simulink subsystem "Luenberger_Tower_FA_Observer"  (R2021a)
settings: Solver=VariableStepAuto  StartTime=0.0  StopTime=10.0  RelTol=1e-3
values from neighbouring files (symbols this model uses):
  Parameters =     [Parameters.mat]
undefined symbols (not defined in the file or in its folder): luenGainDisc1, sys_tower_fa_d_obsv1
libraries: dspstat3 x2
settings Model: Creator=atindriyopamos  LastModifiedBy=zfeng1

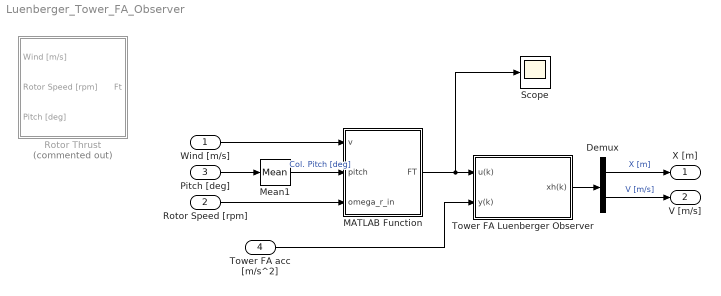
== system Luenberger_Tower_FA_Observer ==
  Wind [m/s] : Inport
  Rotor Speed [rpm] : Inport  Port=2
  Pitch [deg] : Inport  Port=3
  Tower FA acc [m/s^2] : Inport  Port=4
  Demux : Demux  Outputs=2
  MATLAB Function : MATLAB Function  TreatAsAtomicUnit=on
  Mean1 : dspstat3/Mean  run=off  InputProcessing=Columns as channels (frame based)  reset_popup=None  directionMode=Entire input  dimension=1  roiEnable=off  roiType=Rectangles  roiPortion=Entire ROI  roiOutput=Individual statistics for each ROI  roiFlag=off  roundingMode=Floor  overflowMode=off  outputDataTypeStr=Inherit: Same as accumulator  outputMin=[]  outputMax=[]  outputLastDataTypeStr=Inherit: Same as accumulator
  Rotor Thrust : Subsystem  Commented=on
  Scope : Scope
  Tower FA Luenberger Observer : Subsystem
  X [m] : Outport
  V [m/s] : Outport  Port=2
  wires:
  Tower FA acc [m/s^2]/1 -> Tower FA Luenberger Observer/2(y(k))
  Demux/2 -> V [m/s]/1  "V [m/s]"
  Tower FA Luenberger Observer/1(xh(k)) -> Demux/1
  MATLAB Function/1(FT) -> Scope/1, Tower FA Luenberger Observer/1(u(k))
  Wind [m/s]/1 -> MATLAB Function/1(v)
  Rotor Speed [rpm]/1 -> MATLAB Function/3(omega_r_in)
  Demux/1 -> X [m]/1  "X [m]"
  Pitch [deg]/1 -> Mean1/1
  Mean1/1 -> MATLAB Function/2(pitch)  "Col. Pitch [deg]"

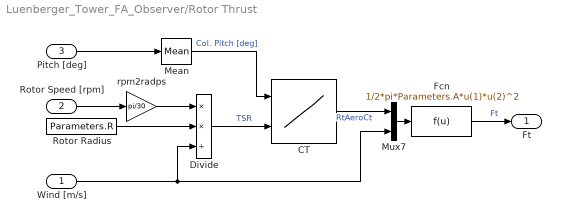
== system Luenberger_Tower_FA_Observer/Rotor Thrust ==
  Wind [m/s] : Inport
  Rotor Speed [rpm] : Inport  Port=2
  Pitch [deg] : Inport  Port=3
  CT : Lookup_n-D  BreakpointsForDimension1=Parameters.Rotor_PitchFull  BreakpointsForDimension2=Parameters.Rotor_Lamda  Table=Parameters.Rotor_cTFull  InternalRulePriority=Speed  RndMeth=Simplest  InputSameDT=on
      settings: InputPortMap=u0,u1
  Divide : Product  Inputs=**/
  Fcn : Fcn  Expr=1/2*pi*Parameters.A*u(1)*u(2)^2
  Mean : dspstat3/Mean  run=off  InputProcessing=Columns as channels (frame based)  reset_popup=None  directionMode=Entire input  dimension=1  roiEnable=off  roiType=Rectangles  roiPortion=Entire ROI  roiOutput=Individual statistics for each ROI  roiFlag=off  roundingMode=Floor  overflowMode=off  outputDataTypeStr=Inherit: Same as accumulator  outputMin=[]  outputMax=[]  outputLastDataTypeStr=Inherit: Same as accumulator
  Mux7 : Mux  Inputs=2
  Rotor Radius : Constant  Value=Parameters.R
  rpm2radps : Gain  Gain=pi/30
  Ft : Outport
  wires:
  Rotor Speed [rpm]/1 -> rpm2radps/1
  Rotor Radius/1 -> Divide/2
  rpm2radps/1 -> Divide/1
  Divide/1 -> CT/2  "TSR"
  Wind [m/s]/1 -> Mux7/2, Divide/3
  Pitch [deg]/1 -> Mean/1
  CT/1 -> Mux7/1  "RtAeroCt"
  Mux7/1 -> Fcn/1
  Mean/1 -> CT/1  "Col. Pitch [deg]"
  Fcn/1 -> Ft/1  "Ft"

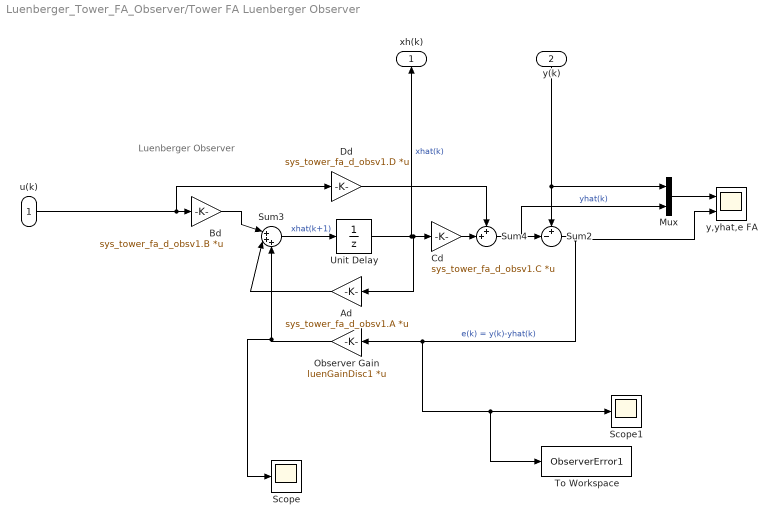
== system Luenberger_Tower_FA_Observer/Tower FA Luenberger Observer ==
  note: Luenberger Observer
  u(k) : Inport
  y(k) : Inport  Port=2
  Ad : Gain  Gain=sys_tower_fa_d_obsv1.A  Multiplication=Matrix(K*u)
  Bd : Gain  Gain=sys_tower_fa_d_obsv1.B  Multiplication=Matrix(K*u)
  Cd : Gain  Gain=sys_tower_fa_d_obsv1.C  Multiplication=Matrix(K*u)
  Dd : Gain  Gain=sys_tower_fa_d_obsv1.D  Multiplication=Matrix(K*u)
  Mux : Mux  Inputs=2
  Observer Gain : Gain  Gain=luenGainDisc1  Multiplication=Matrix(K*u)
  Scope : Scope
  Scope1 : Scope
  Sum2 : Sum  Inputs=+-|
  Sum3 : Sum  Inputs=|+++
  Sum4 : Sum  Inputs=++|
  To Workspace : ToWorkspace  VariableName=ObserverError1  SaveFormat=Timeseries  SampleTime=-1
  Unit Delay : UnitDelay  SampleTime=-1  HasFrameUpgradeWarning=on
  y,yhat,e FA : Scope  NumInputPorts=2
  xh(k) : Outport
  wires:
  Sum2/1 -> Observer Gain/1, Scope1/1, To Workspace/1, y,yhat,e FA/2  "e(k) = y(k)-yhat(k)"
  Sum3/1 -> Unit Delay/1  "xhat(k+1)"
  Cd/1 -> Sum4/2
  Dd/1 -> Sum4/1
  Bd/1 -> Sum3/1
  Observer Gain/1 -> Scope/1, Sum3/3
  Ad/1 -> Sum3/2
  Sum4/1 -> Mux/2, Sum2/2  "yhat(k)"
  y(k)/1 -> Mux/1, Sum2/1
  u(k)/1 -> Dd/1, Bd/1
  Unit Delay/1 -> xh(k)/1, Cd/1, Ad/1  "xhat(k)"
  Mux/1 -> y,yhat,e FA/1

== matlab function Luenberger_Tower_FA_Observer/MATLAB Function ==
  data: v input; FT output; pitch input; omega_r_in input; Parameters parameter
function FT = fcn(v,pitch,omega_r_in,Parameters)

omega_r = omega_r_in *pi/30;
TSR = omega_r*Parameters.R/v;

ct = interp2(Parameters.Rotor_Lamda,Parameters.Rotor_PitchFull,Parameters.Rotor_cTFull,TSR,pitch,'spline');

FT = 1/2*Parameters.rho*pi*Parameters.R^2*ct*v^2;
